simulink model "simulink_control"  (R2024a)
settings: Solver=ode5  StartTime=0.0  StopTime=inf  FixedStep=0.016  RelTol=1e-3
values from neighbouring files (symbols this model uses):
  accelerometer_sensor = wb_robot_get_device('accelerometer')    [simulink_control_app.m]
  gyro_sensor = wb_robot_get_device('gyro')    [simulink_control_app.m]
  left_front_wheel = wb_robot_get_device('left_front_wheel')    [simulink_control_app.m]
  left_rear_wheel = wb_robot_get_device('left_rear_wheel')    [simulink_control_app.m]
  left_steer = wb_robot_get_device('left_steer')    [simulink_control_app.m]
  left_steer_sensor = wb_robot_get_device('left_steer_sensor')    [simulink_control_app.m]
  lidar_sensor = wb_robot_get_device('Sick LMS 291')    [simulink_control_app.m]
  right_front_wheel = wb_robot_get_device('right_front_wheel')    [simulink_control_app.m]
  right_rear_wheel = wb_robot_get_device('right_rear_wheel')    [simulink_control_app.m]
  right_steer = wb_robot_get_device('right_steer')    [simulink_control_app.m]
  right_steer_sensor = wb_robot_get_device('right_steer_sensor')    [simulink_control_app.m]
  TIME_STEP = 16    [simulink_control_app.m]
libraries: eeGeneralControl x2
settings Model: Creator=Harun  LastModifiedBy=Harun

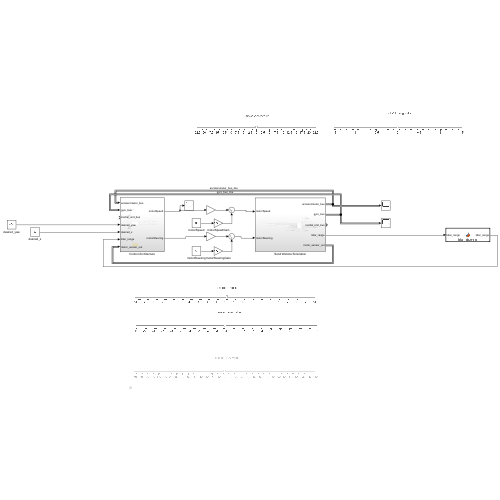
[thumbnail: Simulink's stored preview of the top-level diagram]
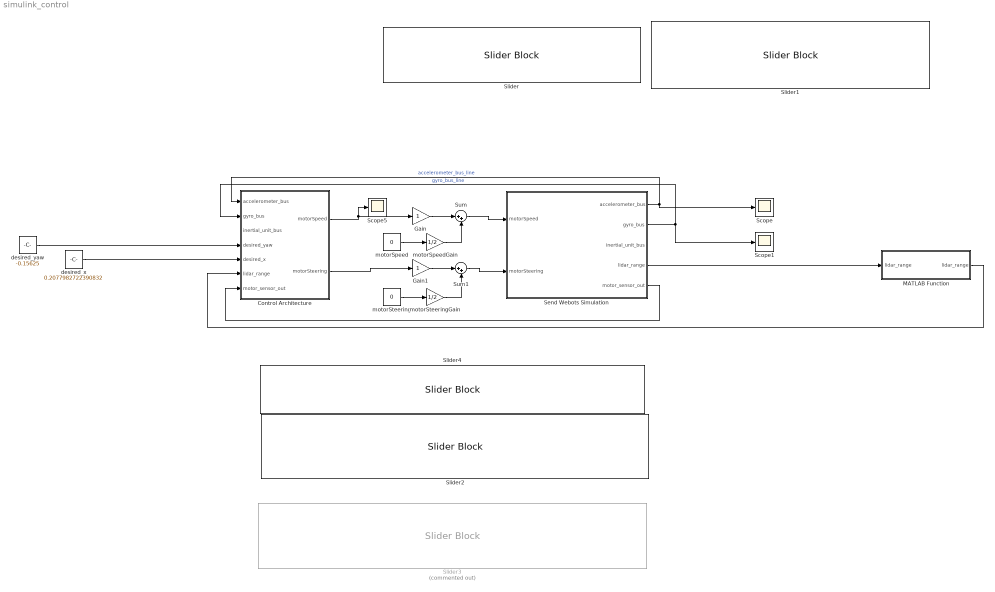
== system simulink_control ==
  Control Architecture : Subsystem
  Gain : Gain
  Gain1 : Gain
  MATLAB Function : MATLAB Function  TreatAsAtomicUnit=on
  Scope : Scope
  Scope1 : Scope
  Scope5 : Scope
  Send Webots Simulation : Subsystem
  Slider : SliderBlock  ScaleMin=-22.5  ScaleMax=22.5  TickInterval=2.5
  Slider1 : SliderBlock  ScaleMin=-1.5  ScaleMax=1.5  TickInterval=0.5
  Slider2 : SliderBlock  ScaleMin=-10  ScaleMax=10  TickInterval=1
  Slider3 : SliderBlock  Commented=on  ScaleMin=-150  ScaleMax=150  TickInterval=10
  Slider4 : SliderBlock  ScaleMin=-10  ScaleMax=10
  Sum : Sum  Inputs=|++
  Sum1 : Sum  Inputs=|++
  desired_x : Constant  Value=0.2077982722390832
  desired_yaw : Constant  Value=-0.15625
  motorSpeed : Constant  Value=0
  motorSpeedGain : Gain  Gain=1/2
  motorSteering : Constant  Value=0
  motorSteeringGain : Gain  Gain=1/2
  wires:
  motorSteering/1 -> motorSteeringGain/1
  motorSpeed/1 -> motorSpeedGain/1
  Sum/1 -> Send Webots Simulation/1(motorSpeed)
  Control Architecture/1(motorSpeed) -> Scope5/1, Gain/1
  Control Architecture/2(motorSteering) -> Gain1/1
  Sum1/1 -> Send Webots Simulation/2(motorSteering)
  motorSpeedGain/1 -> Sum/2
  motorSteeringGain/1 -> Sum1/2
  desired_yaw/1 -> Control Architecture/4(desired_yaw)
  Send Webots Simulation/1(accelerometer_bus) -> Control Architecture/1(accelerometer_bus), Scope/1  "accelerometer_bus_line"
  Send Webots Simulation/2(gyro_bus) -> Control Architecture/2(gyro_bus), Scope1/1  "gyro_bus_line"
  Gain/1 -> Sum/1
  Gain1/1 -> Sum1/1
  desired_x/1 -> Control Architecture/5(desired_x)
  Send Webots Simulation/4(lidar_range) -> MATLAB Function/1("lidar_range ")
  MATLAB Function/1(lidar_range) -> Control Architecture/6(lidar_range)
  Send Webots Simulation/5(motor_sensor_out) -> Control Architecture/7(motor_sensor_out)

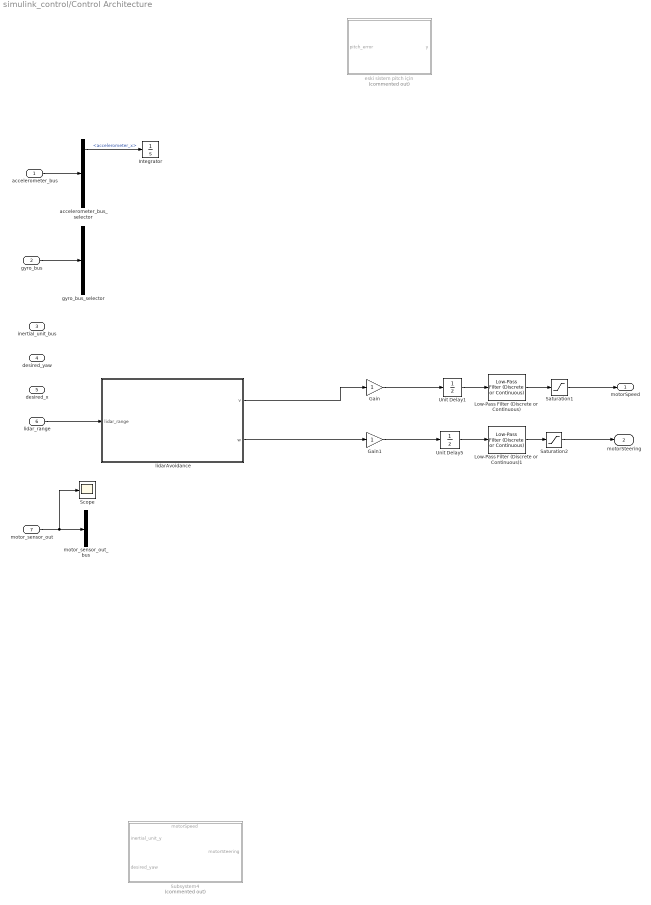
== system simulink_control/Control Architecture ==
  accelerometer_bus : Inport
  gyro_bus : Inport  Port=2
  inertial_unit_bus : Inport  Port=3
  desired_yaw : Inport  Port=4
  desired_x : Inport  Port=5
  lidar_range : Inport  Port=6
  motor_sensor_out : Inport  Port=7
  Gain : Gain
  Gain1 : Gain
  Integrator : Integrator
  Low-Pass Filter (Discrete or Continuous) : eeGeneralControl/Low-Pass Filter (Discrete or Continuous)  K=1  T=0.016  B=inf  A=-inf  init_option=Inherited from block input  x0=0  Ts=-1
  Low-Pass Filter (Discrete or Continuous)1 : eeGeneralControl/Low-Pass Filter (Discrete or Continuous)  K=1  T=0.016  B=inf  A=-inf  init_option=Inherited from block input  x0=0  Ts=-1
  Saturation1 : Saturate  UpperLimit=15  LowerLimit=-15
  Saturation2 : Saturate  UpperLimit=15  LowerLimit=-15
  Scope : Scope
  Subsystem4 : Subsystem  Commented=on
      settings: PortSchema="{\"entries\":[{\"content\":{\"sides\":[{\"content\":{\"connectorIds\":[\"In1\",\"In2\"]},\"type\":\"ConnectorPlacement.EquallySpacedRectSide\",\"uuid\":\"8ea77c90-69e3-4b28-847a-36c3733c4ca1\"},{\"content\":{\"connectorIds\":[\"Out1\"],\"side\":\"RIGHT\"},\"type\":\"ConnectorPlacement.EquallySpacedRectSide\",\"uuid\":\"94f1f4b2-c797-44bf-abc2-6d3fe195cf34\"},{\"content\":{\"connectorIds\":[\"In3\"],\"side\":\"TOP\"},\"type\":\"ConnectorPlacement.EquallySpacedRectSide\",\"uuid\":\"06572095-9567-46cb-bcf7-b6a4abacf0e1\"}]},\"type\":\"ConnectorPlacement.EquallySpacedConnector\",\"uuid\":\"9f096835-0cc4-4d1f-8b4a-1f4eeb97a32d\"}],\"packageUris\":[\"http://schema.mathworks.com/mf0/Connector/R2020b\"],\"version\":\"1.0\"}"
  Unit Delay1 : UnitDelay  SampleTime=-1  HasFrameUpgradeWarning=on
  Unit Delay5 : UnitDelay  SampleTime=-1  HasFrameUpgradeWarning=on
  accelerometer_bus_selector : BusSelector  OutputSignals=accelerometer_x,accelerometer_y,accelerometer_z
  eski sistem pitch için : Subsystem  Commented=on
  gyro_bus_selector : BusSelector  OutputSignals=gyro_x,gyro_y,gyro_z
  lidarAvoidance : MATLAB Function  TreatAsAtomicUnit=on
  motor_sensor_out_bus : BusSelector  OutputSignals=left_steer_sensor_out,right_steer_sensor_out
  motorSpeed : Outport
  motorSteering : Outport  Port=2
  wires:
  accelerometer_bus/1 -> accelerometer_bus_selector/1
  gyro_bus/1 -> gyro_bus_selector/1
  Saturation1/1 -> motorSpeed/1
  Unit Delay1/1 -> Low-Pass Filter (Discrete or Continuous)/1
  Low-Pass Filter (Discrete or Continuous)/1 -> Saturation1/1
  Unit Delay5/1 -> Low-Pass Filter (Discrete or Continuous)1/1
  Low-Pass Filter (Discrete or Continuous)1/1 -> Saturation2/1
  accelerometer_bus_selector/1 -> Integrator/1  "<accelerometer_x>"
  Saturation2/1 -> motorSteering/1
  lidar_range/1 -> lidarAvoidance/1(lidar_range)
  lidarAvoidance/1(v) -> Gain/1
  lidarAvoidance/2(w) -> Gain1/1
  motor_sensor_out/1 -> Scope/1, motor_sensor_out_bus/1
  Gain/1 -> Unit Delay1/1
  Gain1/1 -> Unit Delay5/1

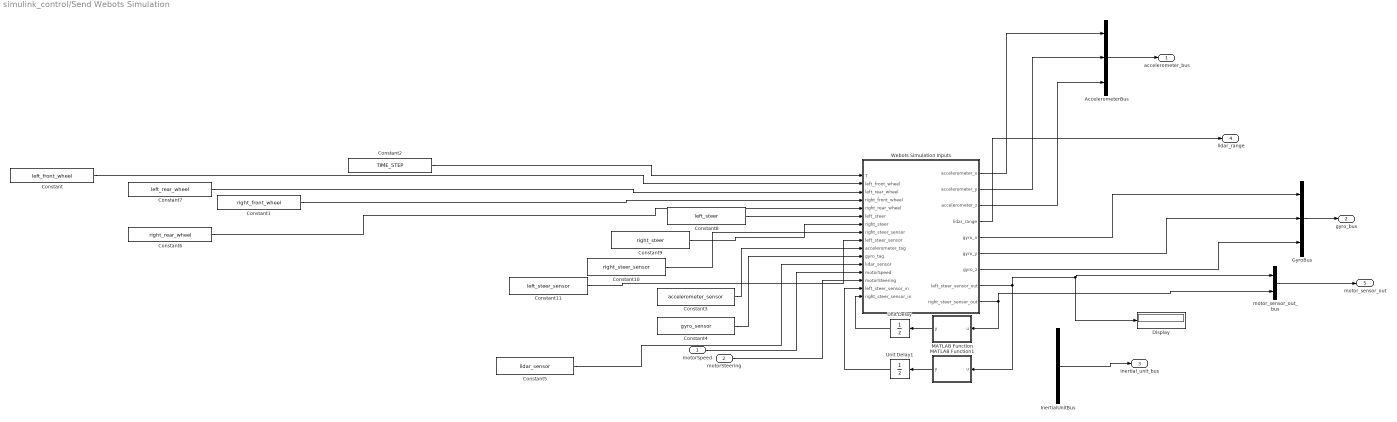
== system simulink_control/Send Webots Simulation ==
  motorSpeed : Inport
  motorSteering : Inport  Port=2
  AccelerometerBus : BusCreator  Inputs=3
  Constant : Constant  Value=left_front_wheel
  Constant1 : Constant  Value=right_front_wheel
  Constant10 : Constant  Value=right_steer_sensor
  Constant11 : Constant  Value=left_steer_sensor
  Constant2 : Constant  Value=TIME_STEP
  Constant3 : Constant  Value=accelerometer_sensor
  Constant4 : Constant  Value=gyro_sensor
  Constant5 : Constant  Value=lidar_sensor
  Constant6 : Constant  Value=right_rear_wheel
  Constant7 : Constant  Value=left_rear_wheel
  Constant8 : Constant  Value=left_steer
  Constant9 : Constant  Value=right_steer
  Display : Display
  GyroBus : BusCreator  Inputs=3
  InertialUnitBus : BusCreator  Inputs=3
  MATLAB Function : MATLAB Function  TreatAsAtomicUnit=on
  MATLAB Function1 : MATLAB Function  TreatAsAtomicUnit=on
  Unit Delay : UnitDelay  SampleTime=-1  HasFrameUpgradeWarning=on
  Unit Delay1 : UnitDelay  SampleTime=-1  HasFrameUpgradeWarning=on
  Webots Simulation Inputs : MATLAB Function  TreatAsAtomicUnit=on
  motor_sensor_out_bus : BusCreator  Inputs=2
  accelerometer_bus : Outport
  gyro_bus : Outport  Port=2
  inertial_unit_bus : Outport  Port=3
  lidar_range : Outport  Port=4
  motor_sensor_out : Outport  Port=5
  wires:
  Constant1/1 -> Webots Simulation Inputs/4(right_front_wheel)
  Constant2/1 -> Webots Simulation Inputs/1(T)
  Constant/1 -> Webots Simulation Inputs/2(left_front_wheel)
  Webots Simulation Inputs/2(accelerometer_y) -> AccelerometerBus/2
  Webots Simulation Inputs/1(accelerometer_x) -> AccelerometerBus/1
  Webots Simulation Inputs/3(accelerometer_z) -> AccelerometerBus/3
  AccelerometerBus/1 -> accelerometer_bus/1
  Constant3/1 -> Webots Simulation Inputs/10(accelerometer_tag)
  Webots Simulation Inputs/7(gyro_z) -> GyroBus/3
  Webots Simulation Inputs/6(gyro_y) -> GyroBus/2
  GyroBus/1 -> gyro_bus/1
  Webots Simulation Inputs/5(gyro_x) -> GyroBus/1
  InertialUnitBus/1 -> inertial_unit_bus/1
  Webots Simulation Inputs/4(lidar_range) -> lidar_range/1
  Webots Simulation Inputs/9(right_steer_sensor_out) -> motor_sensor_out_bus/2, MATLAB Function/1(u)
  motor_sensor_out_bus/1 -> motor_sensor_out/1
  Constant6/1 -> Webots Simulation Inputs/5(right_rear_wheel)
  Constant7/1 -> Webots Simulation Inputs/3(left_rear_wheel)
  MATLAB Function/1(y) -> Unit Delay/1
  MATLAB Function1/1(y) -> Unit Delay1/1
  Webots Simulation Inputs/8(left_steer_sensor_out) -> Display/1, motor_sensor_out_bus/1, MATLAB Function1/1(u)
  Constant4/1 -> Webots Simulation Inputs/11(gyro_tag)
  motorSpeed/1 -> Webots Simulation Inputs/13(motorSpeed)
  motorSteering/1 -> Webots Simulation Inputs/14(motorSteering)
  Unit Delay/1 -> Webots Simulation Inputs/16(right_steer_sensor_in)
  Unit Delay1/1 -> Webots Simulation Inputs/15(left_steer_sensor_in)
  Constant5/1 -> Webots Simulation Inputs/12(lidar_sensor)
  Constant8/1 -> Webots Simulation Inputs/6(left_steer)
  Constant9/1 -> Webots Simulation Inputs/7(right_steer)
  Constant10/1 -> Webots Simulation Inputs/8(right_steer_sensor)
  Constant11/1 -> Webots Simulation Inputs/9(left_steer_sensor)

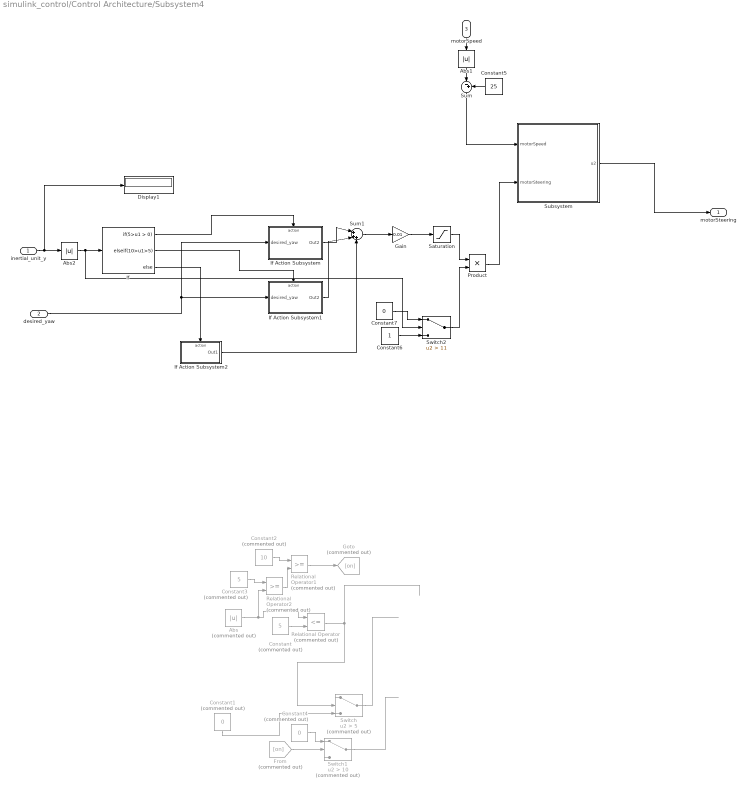
== system simulink_control/Control Architecture/Subsystem4 ==
  inertial_unit_y : Inport
  desired_yaw : Inport  Port=2
  motorSpeed : Inport  Port=3
  Abs : Abs  Commented=on  SaturateOnIntegerOverflow=off
  Abs1 : Abs  SaturateOnIntegerOverflow=off
  Abs2 : Abs  SaturateOnIntegerOverflow=off
  Constant : Constant  Commented=on  Value=5
  Constant1 : Constant  Commented=on  Value=0
  Constant2 : Constant  Commented=on  Value=10
  Constant3 : Constant  Commented=on  Value=5
  Constant4 : Constant  Commented=on  Value=0
  Constant5 : Constant  Value=25
  Constant6 : Constant
  Constant7 : Constant  Value=0
  Display1 : Display
  From : From  Commented=on  GotoTag=on
  Gain : Gain  Gain=0.01
  Goto : Goto  Commented=on  GotoTag=on
  If : If  IfExpression=5>u1 > 0  ElseIfExpressions=10>u1>5
  If Action Subsystem : Subsystem  TreatAsAtomicUnit=on
  If Action Subsystem1 : Subsystem  TreatAsAtomicUnit=on
  If Action Subsystem2 : Subsystem  TreatAsAtomicUnit=on
  Product : Product
  Relational Operator : RelationalOperator  Commented=on  Operator=<=  OutDataTypeStr=boolean  RndMeth=Simplest  InputSameDT=off
  Relational Operator1 : RelationalOperator  Commented=on  OutDataTypeStr=boolean  RndMeth=Simplest  InputSameDT=off
  Relational Operator2 : RelationalOperator  Commented=on  OutDataTypeStr=boolean  RndMeth=Simplest  InputSameDT=off
  Saturation : Saturate  UpperLimit=1000  LowerLimit=-1000
  Subsystem : Subsystem
  Sum : Sum  Inputs=|-+
  Sum1 : Sum  Inputs=|+++
  Switch : Switch  Commented=on  Criteria=u2 > Threshold  Threshold=5  SaturateOnIntegerOverflow=off  InputSameDT=off
  Switch1 : Switch  Commented=on  Criteria=u2 > Threshold  Threshold=10  SaturateOnIntegerOverflow=off  InputSameDT=off
  Switch2 : Switch  Criteria=u2 > Threshold  Threshold=11  SaturateOnIntegerOverflow=off  InputSameDT=off
  motorSteering : Outport
  wires:
  motorSpeed/1 -> Abs1/1
  Abs1/1 -> Sum/1
  Constant5/1 -> Sum/2
  Constant1/1 -> Switch/3
  From/1 -> Switch1/2
  Constant4/1 -> Switch1/1
  Switch1/1 -> ?
  Constant/1 -> Relational Operator/2
  Relational Operator1/1 -> Goto/1
  Constant3/1 -> Relational Operator2/1
  Abs/1 -> Relational Operator2/2, Relational Operator/1
  ? -> Switch1/3, Switch/1
  Constant2/1 -> Relational Operator1/1
  Switch/1 -> ?
  Relational Operator2/1 -> Relational Operator1/2
  Relational Operator/1 -> Switch/2
  inertial_unit_y/1 -> Display1/1, Abs2/1
  If/3 -> If Action Subsystem2/Action
  Abs2/1 -> Switch2/2, If/1
  If/1 -> If Action Subsystem/Action
  If Action Subsystem1/1(Out2) -> Sum1/2
  If Action Subsystem/1(Out2) -> Sum1/1
  If/2 -> If Action Subsystem1/Action
  Sum1/1 -> Gain/1
  Gain/1 -> Saturation/1
  Sum/1 -> Subsystem/1(motorSpeed)
  Saturation/1 -> Product/1
  Constant6/1 -> Switch2/3
  Constant7/1 -> Switch2/1
  Switch2/1 -> Product/2
  Product/1 -> Subsystem/2(motorSteering)
  If Action Subsystem2/1(Out1) -> Sum1/3
  desired_yaw/1 -> If Action Subsystem/1(desired_yaw), If Action Subsystem1/1(desired_yaw)
  Subsystem/1(u2) -> motorSteering/1

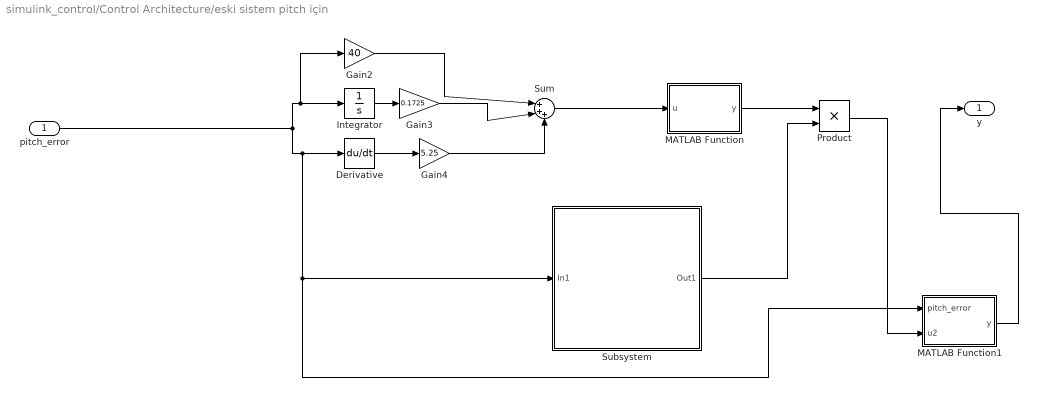
== system simulink_control/Control Architecture/eski sistem pitch için ==
  pitch_error : Inport
  Derivative : Derivative  CoefficientInTFapproximation=0.016
  Gain2 : Gain  Gain=40
  Gain3 : Gain  Gain=0.1725
  Gain4 : Gain  Gain=5.25
  Integrator : Integrator
  MATLAB Function : MATLAB Function  TreatAsAtomicUnit=on
  MATLAB Function1 : MATLAB Function  TreatAsAtomicUnit=on
  Product : Product
  Subsystem : Subsystem
  Sum : Sum  Inputs=|+++
  y : Outport
  wires:
  MATLAB Function1/1(y) -> y/1
  Product/1 -> MATLAB Function1/2(u2)
  MATLAB Function/1(y) -> Product/1
  Sum/1 -> MATLAB Function/1(u)
  Subsystem/1(Out1) -> Product/2
  pitch_error/1 -> Integrator/1, Gain2/1, Derivative/1, MATLAB Function1/1(pitch_error), Subsystem/1(In1)
  Gain4/1 -> Sum/3
  Gain2/1 -> Sum/1
  Gain3/1 -> Sum/2
  Integrator/1 -> Gain3/1
  Derivative/1 -> Gain4/1

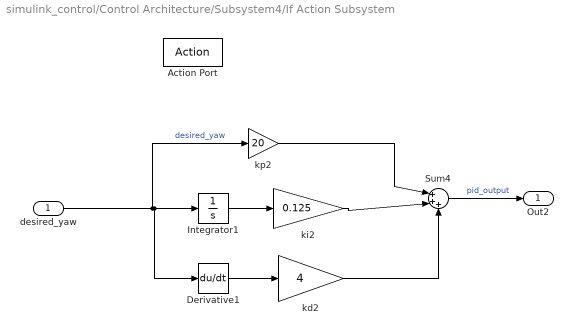
== system simulink_control/Control Architecture/Subsystem4/If Action Subsystem ==
  desired_yaw : Inport
  Action Port : ActionPort
  Derivative1 : Derivative  CoefficientInTFapproximation=0.016
  Integrator1 : Integrator
  Sum4 : Sum  Inputs=|+++
  kd2 : Gain  Gain=4
  ki2 : Gain  Gain=0.125
  kp2 : Gain  Gain=20
  Out2 : Outport
  wires:
  Derivative1/1 -> kd2/1
  Sum4/1 -> Out2/1  "pid_output"
  kp2/1 -> Sum4/1
  ki2/1 -> Sum4/2
  Integrator1/1 -> ki2/1
  desired_yaw/1 -> kp2/1, Derivative1/1, Integrator1/1  "desired_yaw"
  kd2/1 -> Sum4/3

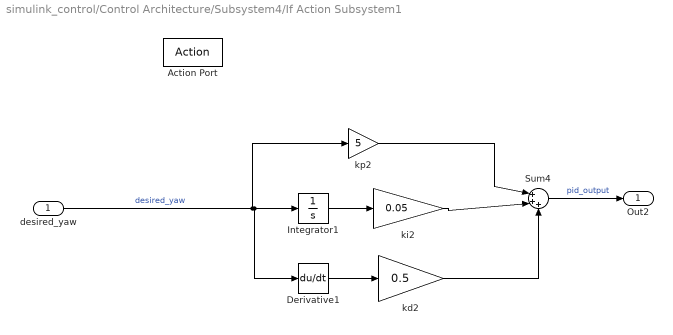
== system simulink_control/Control Architecture/Subsystem4/If Action Subsystem1 ==
  desired_yaw : Inport
  Action Port : ActionPort
  Derivative1 : Derivative  CoefficientInTFapproximation=0.016
  Integrator1 : Integrator
  Sum4 : Sum  Inputs=|+++
  kd2 : Gain  Gain=0.5
  ki2 : Gain  Gain=0.05
  kp2 : Gain  Gain=5
  Out2 : Outport
  wires:
  Derivative1/1 -> kd2/1
  Sum4/1 -> Out2/1  "pid_output"
  kp2/1 -> Sum4/1
  ki2/1 -> Sum4/2
  Integrator1/1 -> ki2/1
  desired_yaw/1 -> kp2/1, Derivative1/1, Integrator1/1  "desired_yaw"
  kd2/1 -> Sum4/3

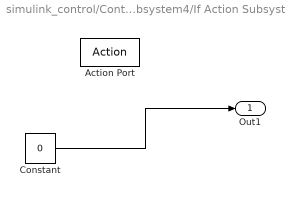
== system simulink_control/Control Architecture/Subsystem4/If Action Subsystem2 ==
  Action Port : ActionPort
  Constant : Constant  Value=0
  Out1 : Outport
  wires:
  Constant/1 -> Out1/1

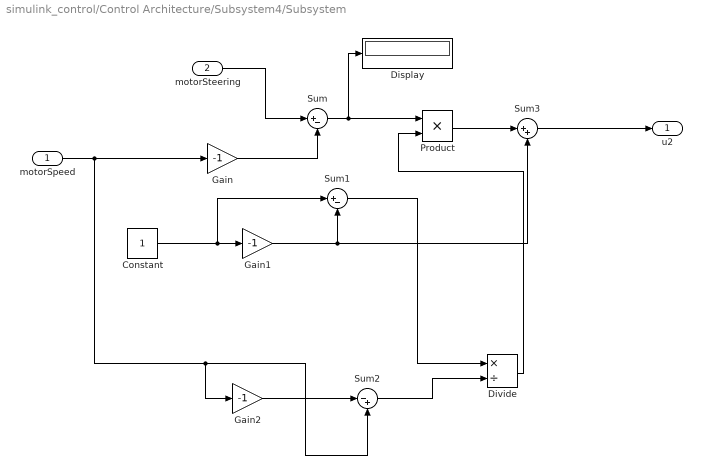
== system simulink_control/Control Architecture/Subsystem4/Subsystem ==
  motorSpeed : Inport
  motorSteering : Inport  Port=2
  Constant : Constant
  Display : Display
  Divide : Product  Inputs=*/
  Gain : Gain  Gain=-1
  Gain1 : Gain  Gain=-1
  Gain2 : Gain  Gain=-1
  Product : Product
  Sum : Sum  Inputs=|+-
  Sum1 : Sum  Inputs=|+-
  Sum2 : Sum  Inputs=|-+
  Sum3 : Sum  Inputs=|++
  u2 : Outport
  wires:
  Sum3/1 -> u2/1
  Product/1 -> Sum3/1
  Divide/1 -> Product/2
  Sum1/1 -> Divide/1
  Sum2/1 -> Divide/2
  Gain2/1 -> Sum2/1
  motorSpeed/1 -> Gain2/1, Sum2/2, Gain/1
  Constant/1 -> Gain1/1, Sum1/1
  Gain1/1 -> Sum1/2, Sum3/2
  Sum/1 -> Display/1, Product/1
  Gain/1 -> Sum/2
  motorSteering/1 -> Sum/1

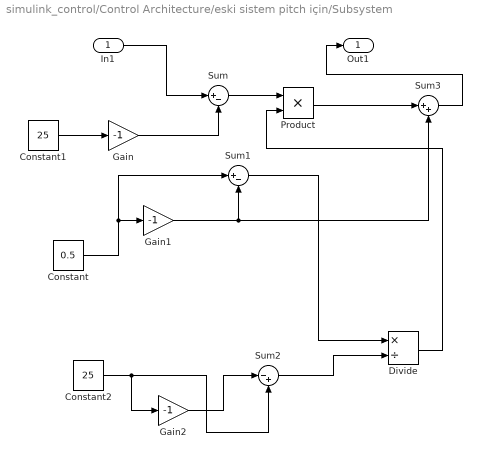
== system simulink_control/Control Architecture/eski sistem pitch için/Subsystem ==
  In1 : Inport
  Constant : Constant  Value=0.5
  Constant1 : Constant  Value=25
  Constant2 : Constant  Value=25
  Divide : Product  Inputs=*/
  Gain : Gain  Gain=-1
  Gain1 : Gain  Gain=-1
  Gain2 : Gain  Gain=-1
  Product : Product
  Sum : Sum  Inputs=|+-
  Sum1 : Sum  Inputs=|+-
  Sum2 : Sum  Inputs=|-+
  Sum3 : Sum  Inputs=|++
  Out1 : Outport
  wires:
  Sum3/1 -> Out1/1
  Product/1 -> Sum3/1
  Divide/1 -> Product/2
  Sum1/1 -> Divide/1
  Sum2/1 -> Divide/2
  Gain2/1 -> Sum2/1
  Constant2/1 -> Gain2/1, Sum2/2
  Constant/1 -> Gain1/1, Sum1/1
  Gain1/1 -> Sum1/2, Sum3/2
  Sum/1 -> Product/1
  Gain/1 -> Sum/2
  Constant1/1 -> Gain/1
  In1/1 -> Sum/1

== matlab function simulink_control/Send Webots Simulation/MATLAB Function1 ==
  data: u input; y output
function y = fcn(u)

y = u;

== matlab function simulink_control/Control Architecture/eski sistem pitch için/MATLAB Function ==
  data: u input; y output
function y = fcn(u)



y = max(-250,min(250,u));
end

== matlab function simulink_control/Control Architecture/eski sistem pitch için/MATLAB Function1 ==
  data: pitch_error input; y output; u2 input
function y = fcn(pitch_error,u2)
if(pitch_error<0)
    y=-u2
else
    y=u2
end

== matlab function simulink_control/MATLAB Function ==
  data: lidar_range input; lidar_range output
function lidar_range =  lidar_showing(lidar_range)
polarplot(lidar_range);
lidar_range=lidar_range;

== matlab function simulink_control/Send Webots Simulation/Webots Simulation Inputs ==
  data: T input; left_front_wheel input; left_rear_wheel input; right_front_wheel input; right_rear_wheel input; left_steer input; accelerometer_x output; accelerometer_y output; accelerometer_z output; lidar_range output; gyro_x output; gyro_y output; gyro_z output; left_steer_sensor_out output; right_steer_sensor_out output; right_steer input; right_steer_sensor input; left_steer_sensor input; accelerometer_tag input; gyro_tag input; lidar_sensor input; motorSpeed input; motorSteering input; left_steer_sensor_in input; right_steer_sensor_in input
function [accelerometer_x,accelerometer_y,accelerometer_z,lidar_range,gyro_x,gyro_y,gyro_z,left_steer_sensor_out,right_steer_sensor_out] = simulation(T ... 
    ,left_front_wheel ,left_rear_wheel,right_front_wheel,right_rear_wheel ...
    , left_steer, right_steer ...
    , right_steer_sensor, left_steer_sensor ...
    , accelerometer_tag,gyro_tag,lidar_sensor ...
    ,motorSpeed,motorSteering,left_steer_sensor_in,right_steer_sensor_in)

accelerometer_x = 0.0;
accelerometer_y = 0.0;
accelerometer_z = 0.0;

gyro_x=0.0;
gyro_y=0.0;
gyro_z=0.0;

wb_robot_step(T)
wb_lidar_enable_point_cloud(lidar_sensor);

% Speed

wb_motor_set_position(left_front_wheel, Inf);
wb_motor_set_position(left_rear_wheel, Inf);
wb_motor_set_position(right_front_wheel,Inf);
wb_motor_set_position(right_rear_wheel,Inf);
wb_motor_set_velocity(left_front_wheel, motorSpeed+motorSteering*0.5);
wb_motor_set_velocity(left_rear_wheel, motorSpeed+motorSteering*0.5);
wb_motor_set_velocity(right_front_wheel,motorSpeed-motorSteering*0.5);
wb_motor_set_velocity(right_rear_wheel,motorSpeed-motorSteering*0.5);

% Steer

wb_motor_set_position(left_steer,motorSteering);
wb_motor_set_position(right_steer,motorSteering);

left_steer_sensor_out=0;
right_steer_sensor_out=0;
left_steer_sensor_out=wb_motor_get_position_sensor(left_steer_sensor);
right_steer_sensor_out=wb_motor_get_position_sensor(right_steer_sensor);

%left_motor_sensor_out=left_motor_sensor_in+left_motor_sensor_out;
%right_motor_sensor_out=left_motor_sensor_in+right_motor_sensor_out;


%period = wb_accelerometer_get_sampling_period(accelerometer_tag)
accelerometer_values = zeros(1, 3); 
accelerometer_values = wb_accelerometer_get_values(accelerometer_tag);
accelerometer_x = accelerometer_values(1);
accelerometer_y = accelerometer_values(2);
accelerometer_z = accelerometer_values(3);

%disp(wb_lidar_get_range_image(lidar_sensor))
lidar_range=zeros(1,180);
lidar_range =double(wb_lidar_get_range_image(lidar_sensor));



gyro_values = zeros(1, 3); 
gyro_values = wb_gyro_get_values(gyro_tag);

gyro_x = gyro_values(1);
gyro_y = gyro_values(2);
gyro_z = gyro_values(3);

end

== matlab function simulink_control/Control Architecture/lidarAvoidance ==
  data: lidar_range input; v output; w output
function [v,w]= lidarAvoidance(lidar_range)
%#codegen
    N= length(lidar_range);
    left_range=lidar_range(1:45);
    front_range=lidar_range(45:135);
    right_range=lidar_range(135:180);
    
    avg_left=mean(left_range(~isinf(left_range)));
    avg_front=mean(front_range(~isinf(front_range)));
    avg_right=mean(right_range(~isinf(right_range)));

    treshold=3.0;
    
    v=2.5;
    w=0.0;
    
    if avg_front<treshold
        if avg_left>avg_right
            v=2.2;
            w=-1.5;

        elseif avg_right>avg_left
            v=2.2;
            w=-1.5;
        else
            v=0.0;
            w=0.0;
        end
    end
end

== matlab function simulink_control/Send Webots Simulation/MATLAB Function ==
  data: u input; y output
function y = fcn(u)

y = u;
